simulink model "DYN_01x"  (R2021a)
settings: Solver=FixedStepAuto  StartTime=0.0  StopTime=50  FixedStep=0.001  RelTol=1e-3
settings Model: Creator=TMP  LastModifiedBy=TMP
settings SolverCC: AlgebraicLoopSolver=TrustRegion
settings DebuggingCC: SFMachineParentedDataDiag=warning

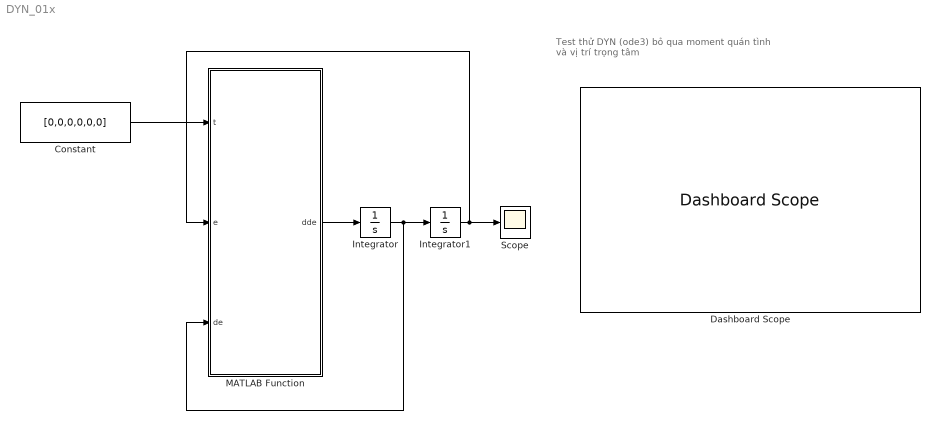
== system DYN_01x ==
  note: Test thử DYN (ode3)
      | bỏ qua moment quán tình và vị trí trọng tâm
  Constant : Constant  Value=[0,0,0,0,0,0]
  Dashboard Scope : DashboardScope
  Integrator : Integrator  InitialCondition=[0.2;0.2;0.2;0.2;0.2;0.2]
  Integrator1 : Integrator  InitialCondition=[0.1;0.1;0.1;0.1;0.1;0.1]
  MATLAB Function : MATLAB Function  TreatAsAtomicUnit=on
  Scope : Scope
  wires:
  MATLAB Function/1(dde) -> Integrator/1
  Integrator/1 -> Integrator1/1, MATLAB Function/3(de)
  Integrator1/1 -> Scope/1, MATLAB Function/2(e)
  Constant/1 -> MATLAB Function/1(t)

== matlab function DYN_01x/MATLAB Function ==
  data: t input; e input; dde output; de input
function dde = fcn(t,e,de)
e1 = e(1); e2 = e(2); e3 = e(3);
e4 = e(4); e5 = e(5); e6 = e(6);
de1 = de(1); de2 = de(2); de3 = de(3);
de4 = de(4); de5 = de(5); de6 = de(6);
g = 9.81;
a1=0.75; a2=2.70; a3=0.90; d1=3.35; d4=2.95; d7=0.80;
I1=0; I2=0; I3=0; I4=0; I5=0; I6=0.1;
m1 = 5.6511; m2 = 4.6061; m3 = 4.2963; m4 = 1.9151; m5 = 0.3399; m6 = 0.0714;

M = [I1 + I2 + I3 + I4 + I5 + I6 + a1^2*m2 + a1^2*m3 + a1^2*m4 + (a2^2*m3)/2 + a1^2*m5 + (a2^2*m4)/2 + a1^2*m6 + (a2^2*m5)/2 + (a3^2*m4)/2 + (a2^2*m6)/2 + (a3^2*m5)/2 + (a3^2*m6)/2 + (d4^2*m4)/2 + (d4^2*m5)/2 + (d4^2*m6)/2 - (a2^2*m3*cos(2*e2))/2 - (a2^2*m4*cos(2*e2))/2 - (a2^2*m5*cos(2*e2))/2 - (a2^2*m6*cos(2*e2))/2 - (a3^2*m4*cos(2*e2 + 2*e3))/2 - (a3^2*m5*cos(2*e2 + 2*e3))/2 - (a3^2*m6*cos(2*e2 + 2*e3))/2 + (d4^2*m4*cos(2*e2 + 2*e3))/2 + (d4^2*m5*cos(2*e2 + 2*e3))/2 + (d4^2*m6*cos(2*e2 + 2*e3))/2 + 2*a1*d4*m4*cos(e2 + e3) + 2*a1*d4*m5*cos(e2 + e3) + 2*a1*d4*m6*cos(e2 + e3) + 2*a1*a3*m4*sin(e2 + e3) + 2*a1*a3*m5*sin(e2 + e3) + 2*a1*a3*m6*sin(e2 + e3) + a2*a3*m4*cos(e3) + a2*a3*m5*cos(e3) + a2*a3*m6*cos(e3) + 2*a1*a2*m3*sin(e2) + 2*a1*a2*m4*sin(e2) + 2*a1*a2*m5*sin(e2) + 2*a1*a2*m6*sin(e2) - a2*d4*m4*sin(e3) - a2*d4*m5*sin(e3) - a2*d4*m6*sin(e3) - a2*a3*m4*cos(2*e2 + e3) - a2*a3*m5*cos(2*e2 + e3) - a2*a3*m6*cos(2*e2 + e3) + a2*d4*m4*sin(2*e2 + e3) + a2*d4*m5*sin(2*e2 + e3) + a2*d4*m6*sin(2*e2 + e3) + a3*d4*m4*sin(2*e2 + 2*e3) + a3*d4*m5*sin(2*e2 + 2*e3) + a3*d4*m6*sin(2*e2 + 2*e3),0,0,-sin(e2 + e3)*(I4 + I5 + I6),cos(e2 + e3)*sin(e4)*(I5 + I6),I6*cos(e4)*sin(e2)*sin(e3)*sin(e5) - I6*cos(e3)*cos(e5)*sin(e2) - I6*cos(e2)*cos(e3)*cos(e4)*sin(e5) - I6*cos(e2)*cos(e5)*sin(e3);
     0,I2 + I3 + I4 + I5 + I6 + a2^2*m3 + a2^2*m4 + a2^2*m5 + a3^2*m4 + a2^2*m6 + a3^2*m5 + a3^2*m6 + d4^2*m4 + d4^2*m5 + d4^2*m6 + 2*a2*a3*m4*cos(e3) + 2*a2*a3*m5*cos(e3) + 2*a2*a3*m6*cos(e3) - 2*a2*d4*m4*sin(e3) - 2*a2*d4*m5*sin(e3) - 2*a2*d4*m6*sin(e3),I3 + I4 + I5 + I6 + a3^2*m4 + a3^2*m5 + a3^2*m6 + d4^2*m4 + d4^2*m5 + d4^2*m6 + a2*a3*m4*cos(e3) + a2*a3*m5*cos(e3) + a2*a3*m6*cos(e3) - a2*d4*m4*sin(e3) - a2*d4*m5*sin(e3) - a2*d4*m6*sin(e3),0,cos(e4)*(I5 + I6),I6*sin(e4)*sin(e5);
     0,I3 + I4 + I5 + I6 + a3^2*m4 + a3^2*m5 + a3^2*m6 + d4^2*m4 + d4^2*m5 + d4^2*m6 + a2*a3*m4*cos(e3) + a2*a3*m5*cos(e3) + a2*a3*m6*cos(e3) - a2*d4*m4*sin(e3) - a2*d4*m5*sin(e3) - a2*d4*m6*sin(e3),I3 + I4 + I5 + I6 + a3^2*m4 + a3^2*m5 + a3^2*m6 + d4^2*m4 + d4^2*m5 + d4^2*m6,0,cos(e4)*(I5 + I6),I6*sin(e4)*sin(e5);
    -sin(e2 + e3)*(I4 + I5 + I6),0,0,I4 + I5 + I6,0,I6*cos(e5);
    cos(e2 + e3)*sin(e4)*(I5 + I6),cos(e4)*(I5 + I6),cos(e4)*(I5 + I6),0,I5 + I6,0;
    I6*cos(e4)*sin(e2)*sin(e3)*sin(e5) - I6*cos(e3)*cos(e5)*sin(e2) - I6*cos(e2)*cos(e3)*cos(e4)*sin(e5) - I6*cos(e2)*cos(e5)*sin(e3),I6*sin(e4)*sin(e5),I6*sin(e4)*sin(e5),I6*cos(e5),0,I6];

C = ...
[de2*(a2^2*m3*sin(2*e2) + a2^2*m4*sin(2*e2) + a2^2*m5*sin(2*e2) + a2^2*m6*sin(2*e2) + a3^2*m4*sin(2*e2 + 2*e3) + a3^2*m5*sin(2*e2 + 2*e3) + a3^2*m6*sin(2*e2 + 2*e3) - d4^2*m4*sin(2*e2 + 2*e3) - d4^2*m5*sin(2*e2 + 2*e3) - d4^2*m6*sin(2*e2 + 2*e3) + 2*a1*a3*m4*cos(e2 + e3) + 2*a1*a3*m5*cos(e2 + e3) + 2*a1*a3*m6*cos(e2 + e3) - 2*a1*d4*m4*sin(e2 + e3) - 2*a1*d4*m5*sin(e2 + e3) - 2*a1*d4*m6*sin(e2 + e3) + 2*a1*a2*m3*cos(e2) + 2*a1*a2*m4*cos(e2) + 2*a1*a2*m5*cos(e2) + 2*a1*a2*m6*cos(e2) + 2*a2*d4*m4*cos(2*e2 + e3) + 2*a2*d4*m5*cos(2*e2 + e3) + 2*a2*d4*m6*cos(2*e2 + e3) + 2*a2*a3*m4*sin(2*e2 + e3) + 2*a2*a3*m5*sin(2*e2 + e3) + 2*a2*a3*m6*sin(2*e2 + e3) + 2*a3*d4*m4*cos(2*e2 + 2*e3) + 2*a3*d4*m5*cos(2*e2 + 2*e3) + 2*a3*d4*m6*cos(2*e2 + 2*e3)) + de3*(m4 + m5 + m6)*(a3^2*sin(2*e2 + 2*e3) - d4^2*sin(2*e2 + 2*e3) + a2*d4*cos(2*e2 + e3) + a2*a3*sin(2*e2 + e3) + 2*a3*d4*cos(2*e2 + 2*e3) + 2*a1*a3*cos(e2 + e3) - 2*a1*d4*sin(e2 + e3) - a2*d4*cos(e3) - a2*a3*sin(e3)),0,0,-cos(e2 + e3)*(de2 + de3)*(I4 + I5 + I6),-(I5 + I6)*(de2*sin(e2 + e3)*sin(e4) - de4*cos(e2 + e3)*cos(e4) + de3*sin(e2 + e3)*sin(e4)),I6*de2*(cos(e5)*sin(e2)*sin(e3) - cos(e2)*cos(e3)*cos(e5) + cos(e2)*cos(e4)*sin(e3)*sin(e5) + cos(e3)*cos(e4)*sin(e2)*sin(e5)) + I6*de3*(cos(e5)*sin(e2)*sin(e3) - cos(e2)*cos(e3)*cos(e5) + cos(e2)*cos(e4)*sin(e3)*sin(e5) + cos(e3)*cos(e4)*sin(e2)*sin(e5)) + I6*de5*(cos(e2)*sin(e3)*sin(e5) + cos(e3)*sin(e2)*sin(e5) - cos(e2)*cos(e3)*cos(e4)*cos(e5) + cos(e4)*cos(e5)*sin(e2)*sin(e3)) + I6*de4*cos(e2 + e3)*sin(e4)*sin(e5);
 (I4*de4*cos(e2 + e3))/2 + (I5*de4*cos(e2 + e3))/2 + (I6*de4*cos(e2 + e3))/2 - (a2^2*de1*m3*sin(2*e2))/2 - (a2^2*de1*m4*sin(2*e2))/2 - (a2^2*de1*m5*sin(2*e2))/2 - (a2^2*de1*m6*sin(2*e2))/2 - (a3^2*de1*m4*sin(2*e2 + 2*e3))/2 - (a3^2*de1*m5*sin(2*e2 + 2*e3))/2 - (a3^2*de1*m6*sin(2*e2 + 2*e3))/2 + (d4^2*de1*m4*sin(2*e2 + 2*e3))/2 + (d4^2*de1*m5*sin(2*e2 + 2*e3))/2 + (d4^2*de1*m6*sin(2*e2 + 2*e3))/2 + (I5*de5*sin(e2 + e3)*sin(e4))/2 + (I6*de5*sin(e2 + e3)*sin(e4))/2 - a3*d4*de1*m4*cos(2*e2 + 2*e3) - a3*d4*de1*m5*cos(2*e2 + 2*e3) - a3*d4*de1*m6*cos(2*e2 + 2*e3) + (I6*de6*cos(e2)*cos(e3)*cos(e5))/2 - a1*a3*de1*m4*cos(e2 + e3) - a1*a3*de1*m5*cos(e2 + e3) - a1*a3*de1*m6*cos(e2 + e3) - (I6*de6*cos(e5)*sin(e2)*sin(e3))/2 + a1*d4*de1*m4*sin(e2 + e3) + a1*d4*de1*m5*sin(e2 + e3) + a1*d4*de1*m6*sin(e2 + e3) - a1*a2*de1*m3*cos(e2) - a1*a2*de1*m4*cos(e2) - a1*a2*de1*m5*cos(e2) - a1*a2*de1*m6*cos(e2) - a2*d4*de1*m4*cos(2*e2 + e3) - a2*d4*de1*m5*cos(2*e2 + e3) - a2*d4*de1*m6*cos(2*e2 + e3) - a2*a3*de1*m4*sin(2*e2 + e3) - a2*a3*de1*m5*sin(2*e2 + e3) - a2*a3*de1*m6*sin(2*e2 + e3) - (I6*de6*cos(e2)*cos(e4)*sin(e3)*sin(e5))/2 - (I6*de6*cos(e3)*cos(e4)*sin(e2)*sin(e5))/2,-2*a2*de3*(d4*cos(e3) + a3*sin(e3))*(m4 + m5 + m6),-a2*de3*(d4*cos(e3) + a3*sin(e3))*(m4 + m5 + m6),(de1*cos(e2 + e3)*(I4 + I5 + I6))/2,-(sin(e4)*(2*de4 - de1*sin(e2 + e3))*(I5 + I6))/2,(I6*(2*de4*cos(e4)*sin(e5) + 2*de5*cos(e5)*sin(e4) + de1*cos(e2)*cos(e3)*cos(e5) - de1*cos(e5)*sin(e2)*sin(e3) - de1*cos(e2)*cos(e4)*sin(e3)*sin(e5) - de1*cos(e3)*cos(e4)*sin(e2)*sin(e5)))/2;
 (de4*cos(e2 + e3)*(I4 + I5 + I6))/2 - (I6*de6*(cos(e5)*sin(e2)*sin(e3) - cos(e2)*cos(e3)*cos(e5) + cos(e2)*cos(e4)*sin(e3)*sin(e5) + cos(e3)*cos(e4)*sin(e2)*sin(e5)))/2 - (de1*(m4 + m5 + m6)*(a3^2*sin(2*e2 + 2*e3) - d4^2*sin(2*e2 + 2*e3) + a2*d4*cos(2*e2 + e3) + a2*a3*sin(2*e2 + e3) + 2*a3*d4*cos(2*e2 + 2*e3) + 2*a1*a3*cos(e2 + e3) - 2*a1*d4*sin(e2 + e3) - a2*d4*cos(e3) - a2*a3*sin(e3)))/2 + (de5*sin(e2 + e3)*sin(e4)*(I5 + I6))/2,(a2*(d4*cos(e3) + a3*sin(e3))*(2*de2 - de3)*(m4 + m5 + m6))/2,(a2*de2*(d4*cos(e3) + a3*sin(e3))*(m4 + m5 + m6))/2,(de1*cos(e2 + e3)*(I4 + I5 + I6))/2,-(sin(e4)*(2*de4 - de1*sin(e2 + e3))*(I5 + I6))/2,(I6*(2*de4*cos(e4)*sin(e5) + 2*de5*cos(e5)*sin(e4) + de1*cos(e2)*cos(e3)*cos(e5) - de1*cos(e5)*sin(e2)*sin(e3) - de1*cos(e2)*cos(e4)*sin(e3)*sin(e5) - de1*cos(e3)*cos(e4)*sin(e2)*sin(e5)))/2;
 - cos(e2 + e3)*(de2 + de3)*(I4 + I5 + I6) - (de5*cos(e2 + e3)*cos(e4)*(I5 + I6))/2 - (I6*de6*cos(e2 + e3)*sin(e4)*sin(e5))/2,(de5*sin(e4)*(I5 + I6))/2 - (I6*de6*cos(e4)*sin(e5))/2,(de5*sin(e4)*(I5 + I6))/2 - (I6*de6*cos(e4)*sin(e5))/2,0,((I5 + I6)*(de2*sin(e4) + de3*sin(e4) - de1*cos(e2 + e3)*cos(e4)))/2,-(I6*sin(e5)*(2*de5 + de2*cos(e4) + de3*cos(e4) + de1*cos(e2 + e3)*sin(e4)))/2;
 - (I5 + I6)*(de2*sin(e2 + e3)*sin(e4) - de4*cos(e2 + e3)*cos(e4) + de3*sin(e2 + e3)*sin(e4)) - (I6*de6*(cos(e2)*sin(e3)*sin(e5) + cos(e3)*sin(e2)*sin(e5) - cos(e2)*cos(e3)*cos(e4)*cos(e5) + cos(e4)*cos(e5)*sin(e2)*sin(e3)))/2,- de4*sin(e4)*(I5 + I6) - (I6*de6*cos(e5)*sin(e4))/2,- de4*sin(e4)*(I5 + I6) - (I6*de6*cos(e5)*sin(e4))/2,(I6*de6*sin(e5))/2,0,-(I6*(de2*cos(e5)*sin(e4) - de4*sin(e5) + de3*cos(e5)*sin(e4) + de1*cos(e2)*sin(e3)*sin(e5) + de1*cos(e3)*sin(e2)*sin(e5) + de1*cos(e4)*cos(e5)*sin(e2)*sin(e3) - de1*cos(e2)*cos(e3)*cos(e4)*cos(e5)))/2;
 I6*de2*(cos(e5)*sin(e2)*sin(e3) - cos(e2)*cos(e3)*cos(e5) + cos(e2)*cos(e4)*sin(e3)*sin(e5) + cos(e3)*cos(e4)*sin(e2)*sin(e5)) + I6*de3*(cos(e5)*sin(e2)*sin(e3) - cos(e2)*cos(e3)*cos(e5) + cos(e2)*cos(e4)*sin(e3)*sin(e5) + cos(e3)*cos(e4)*sin(e2)*sin(e5)) + I6*de5*(cos(e2)*sin(e3)*sin(e5) + cos(e3)*sin(e2)*sin(e5) - cos(e2)*cos(e3)*cos(e4)*cos(e5) + cos(e4)*cos(e5)*sin(e2)*sin(e3)) + I6*de4*cos(e2 + e3)*sin(e4)*sin(e5),I6*de4*cos(e4)*sin(e5) + I6*de5*cos(e5)*sin(e4),I6*de4*cos(e4)*sin(e5) + I6*de5*cos(e5)*sin(e4),-I6*de5*sin(e5),0,0];

G = ...
[    
                                                                                                                                                                                              0;
g*(a2*m3*sin(e2) + a2*m4*sin(e2) + a2*m5*sin(e2) + a2*m6*sin(e2) + d4*m4*cos(e2 + e3) + d4*m5*cos(e2 + e3) + d4*m6*cos(e2 + e3) + a3*m4*sin(e2 + e3) + a3*m5*sin(e2 + e3) + a3*m6*sin(e2 + e3));
                                                                                                                                           g*(d4*cos(e2 + e3) + a3*sin(e2 + e3))*(m4 + m5 + m6);
                                                                                                                                                                                              0;
                                                                                                                                                                                              0;
                                                                                                                                                                                              0];
J = ...
[ d4*sin(e1)*sin(e2)*sin(e3) - a2*sin(e1)*sin(e2) - d4*cos(e2)*cos(e3)*sin(e1) - a3*cos(e2)*sin(e1)*sin(e3) - a3*cos(e3)*sin(e1)*sin(e2) - d7*cos(e1)*sin(e4)*sin(e5) - a1*sin(e1) - d7*cos(e2)*cos(e3)*cos(e5)*sin(e1) + d7*cos(e5)*sin(e1)*sin(e2)*sin(e3) + d7*cos(e2)*cos(e4)*sin(e1)*sin(e3)*sin(e5) + d7*cos(e3)*cos(e4)*sin(e1)*sin(e2)*sin(e5), -cos(e1)*(d4*cos(e2)*sin(e3) - a3*cos(e2)*cos(e3) - a2*cos(e2) + d4*cos(e3)*sin(e2) + a3*sin(e2)*sin(e3) + d7*cos(e2)*cos(e5)*sin(e3) + d7*cos(e3)*cos(e5)*sin(e2) + d7*cos(e2)*cos(e3)*cos(e4)*sin(e5) - d7*cos(e4)*sin(e2)*sin(e3)*sin(e5)), -cos(e1)*(d4*cos(e2)*sin(e3) - a3*cos(e2)*cos(e3) + d4*cos(e3)*sin(e2) + a3*sin(e2)*sin(e3) + d7*cos(e2)*cos(e5)*sin(e3) + d7*cos(e3)*cos(e5)*sin(e2) + d7*cos(e2)*cos(e3)*cos(e4)*sin(e5) - d7*cos(e4)*sin(e2)*sin(e3)*sin(e5)), d7*sin(e5)*(cos(e1)*cos(e2)*sin(e3)*sin(e4) - cos(e4)*sin(e1) + cos(e1)*cos(e3)*sin(e2)*sin(e4)), d7*cos(e1)*sin(e2)*sin(e3)*sin(e5) - d7*cos(e1)*cos(e2)*cos(e3)*sin(e5) - d7*cos(e5)*sin(e1)*sin(e4) - d7*cos(e1)*cos(e2)*cos(e4)*cos(e5)*sin(e3) - d7*cos(e1)*cos(e3)*cos(e4)*cos(e5)*sin(e2),                                                                                                                            0;
  a1*cos(e1) + a2*cos(e1)*sin(e2) + d4*cos(e1)*cos(e2)*cos(e3) + a3*cos(e1)*cos(e2)*sin(e3) + a3*cos(e1)*cos(e3)*sin(e2) - d4*cos(e1)*sin(e2)*sin(e3) - d7*sin(e1)*sin(e4)*sin(e5) + d7*cos(e1)*cos(e2)*cos(e3)*cos(e5) - d7*cos(e1)*cos(e5)*sin(e2)*sin(e3) - d7*cos(e1)*cos(e2)*cos(e4)*sin(e3)*sin(e5) - d7*cos(e1)*cos(e3)*cos(e4)*sin(e2)*sin(e5), -sin(e1)*(d4*cos(e2)*sin(e3) - a3*cos(e2)*cos(e3) - a2*cos(e2) + d4*cos(e3)*sin(e2) + a3*sin(e2)*sin(e3) + d7*cos(e2)*cos(e5)*sin(e3) + d7*cos(e3)*cos(e5)*sin(e2) + d7*cos(e2)*cos(e3)*cos(e4)*sin(e5) - d7*cos(e4)*sin(e2)*sin(e3)*sin(e5)), -sin(e1)*(d4*cos(e2)*sin(e3) - a3*cos(e2)*cos(e3) + d4*cos(e3)*sin(e2) + a3*sin(e2)*sin(e3) + d7*cos(e2)*cos(e5)*sin(e3) + d7*cos(e3)*cos(e5)*sin(e2) + d7*cos(e2)*cos(e3)*cos(e4)*sin(e5) - d7*cos(e4)*sin(e2)*sin(e3)*sin(e5)), d7*sin(e5)*(cos(e1)*cos(e4) + cos(e2)*sin(e1)*sin(e3)*sin(e4) + cos(e3)*sin(e1)*sin(e2)*sin(e4)), d7*cos(e1)*cos(e5)*sin(e4) - d7*cos(e2)*cos(e3)*sin(e1)*sin(e5) + d7*sin(e1)*sin(e2)*sin(e3)*sin(e5) - d7*cos(e2)*cos(e4)*cos(e5)*sin(e1)*sin(e3) - d7*cos(e3)*cos(e4)*cos(e5)*sin(e1)*sin(e2),                                                                                                                            0;
                                                                                                                                                                                                                                                                                                                                                     0,            d4*sin(e2)*sin(e3) - d4*cos(e2)*cos(e3) - a3*cos(e2)*sin(e3) - a3*cos(e3)*sin(e2) - a2*sin(e2) - d7*cos(e2)*cos(e3)*cos(e5) + d7*cos(e5)*sin(e2)*sin(e3) + d7*cos(e2)*cos(e4)*sin(e3)*sin(e5) + d7*cos(e3)*cos(e4)*sin(e2)*sin(e5),            d4*sin(e2)*sin(e3) - a3*cos(e2)*sin(e3) - a3*cos(e3)*sin(e2) - d4*cos(e2)*cos(e3) - d7*cos(e2)*cos(e3)*cos(e5) + d7*cos(e5)*sin(e2)*sin(e3) + d7*cos(e2)*cos(e4)*sin(e3)*sin(e5) + d7*cos(e3)*cos(e4)*sin(e2)*sin(e5),                                                                  d7*cos(e2 + e3)*sin(e4)*sin(e5),                                                              d7*cos(e2)*sin(e3)*sin(e5) + d7*cos(e3)*sin(e2)*sin(e5) - d7*cos(e2)*cos(e3)*cos(e4)*cos(e5) + d7*cos(e4)*cos(e5)*sin(e2)*sin(e3),                                                                                                                            0;
                                                                                                                                                                                                                                                                                                                                                     0,                                                                                                                                                                                                                                      -sin(e1),                                                                                                                                                                                                                         -sin(e1),                                                                             cos(e2 + e3)*cos(e1),                                                                                                            cos(e1)*cos(e2)*sin(e3)*sin(e4) - cos(e4)*sin(e1) + cos(e1)*cos(e3)*sin(e2)*sin(e4), cos(e2 + e3)*cos(e1)*cos(e5) - sin(e5)*(sin(e1)*sin(e4) + cos(e1)*cos(e2)*cos(e4)*sin(e3) + cos(e1)*cos(e3)*cos(e4)*sin(e2));
                                                                                                                                                                                                                                                                                                                                                     0,                                                                                                                                                                                                                                       cos(e1),                                                                                                                                                                                                                          cos(e1),                                                                             cos(e2 + e3)*sin(e1),                                                                                                            cos(e1)*cos(e4) + cos(e2)*sin(e1)*sin(e3)*sin(e4) + cos(e3)*sin(e1)*sin(e2)*sin(e4), cos(e2 + e3)*cos(e5)*sin(e1) - sin(e5)*(cos(e2)*cos(e4)*sin(e1)*sin(e3) - cos(e1)*sin(e4) + cos(e3)*cos(e4)*sin(e1)*sin(e2));
                                                                                                                                                                                                                                                                                                                                                     1,                                                                                                                                                                                                                                             0,                                                                                                                                                                                                                                0,                                                                                    -sin(e2 + e3),                                                                                                                                                                           cos(e2 + e3)*sin(e4),                                                                        - sin(e2 + e3)*cos(e5) - cos(e2 + e3)*cos(e4)*sin(e5)];
%%
% V = [V1+5*dt1;V2+5*dt2;V3+5*dt3];
de = [de1;de2;de3;de4;de5;de6];
% V = C*de;
% M_inv = inv(M);
c = 0;
b = 5;
Fe = 0.01*[1;1;1;1;1;1];
F = c*sign(de) + b*de + J'*Fe ;
dde = M\(t-C*de-G-F);
